simulink model "asbQuadcopters_SiFi"  (Simulink 9.1)
settings: Solver=VariableStepAuto  StartTime=0.0  StopTime=TFinal  RelTol=1e-3
values from neighbouring files (symbols this model uses):
  Controller =     [data_set.mat]
  Estimator =     [data_set.mat]
  g = 9.81    [data_set.mat]
  init =     [data_set.mat]
  rho = 1.184    [data_set.mat]
  sensorCalibrationData = [0.09 -0.06 -9.473 -0.0095 -0.0075 0.0015 101270.95 0.2]    [data_set.mat]
  Sensors =     [data_set.mat]
  States =     [data_set.mat]
  takeOffDuration = 1    [data_set.mat]
  Ts = 0.005    [data_set.mat]
  Vehicle =     [data_set.mat]
undefined symbols (not defined in the file or in its folder): DiscIntNeverNeededParam, Discrete, Earth, ft, m, s, sigbuilder_block, Time, WGS84
libraries: simulink x39, aerolibconvert2 x4, sharedutil x3, ctrlSharedLib x3, sharedtransform x3, shared6dof x1, aerolibasang x1, aerolibtransform2 x1, aerolibnav x1, aerolibanimutils x1
(part 2 of 3)

== system asbQuadcopters_SiFi/FCS/State Estimator/EstimatorXYPosition ==
  opticalFlow_datin : Inport
  controlModePosVSOrient_flagin : Inport  Port=2
  usePosVIS_flagin : Inport  Port=3
  posVIS_datin : Inport  Port=4
  sensorIMU_datin : Inport  Port=5
  Z_estimin : Inport  Port=6
  dz_estimin : Inport  Port=7
  orient_estimin : Inport  Port=8
  EstimatorVelocity : Subsystem
  EstimatorXYPosition : Subsystem
  XY_estimout : Outport
  dxy_estimout : Outport  Port=2
  wires:
  EstimatorXYPosition/1(XY_estimout) -> XY_estimout/1
  usePosVIS_flagin/1 -> EstimatorXYPosition/6(usePosVIS_flagin)
  posVIS_datin/1 -> EstimatorXYPosition/5(posVIS_datin)
  dz_estimin/1 -> EstimatorXYPosition/4(dz_estimin)
  controlModePosVSOrient_flagin/1 -> EstimatorXYPosition/3(controlModePosVSOrient_flagin)
  Z_estimin/1 -> EstimatorVelocity/2(Z_estimin)
  sensorIMU_datin/1 -> EstimatorVelocity/3(sensorIMU_datin)
  opticalFlow_datin/1 -> EstimatorVelocity/1(opticalFlow_datin)
  EstimatorVelocity/1(dxy_estimout) -> dxy_estimout/1, EstimatorXYPosition/1(dxy_estimin)
  orient_estimin/1 -> EstimatorXYPosition/2(orient_estimin), EstimatorVelocity/4(orient_estimin)

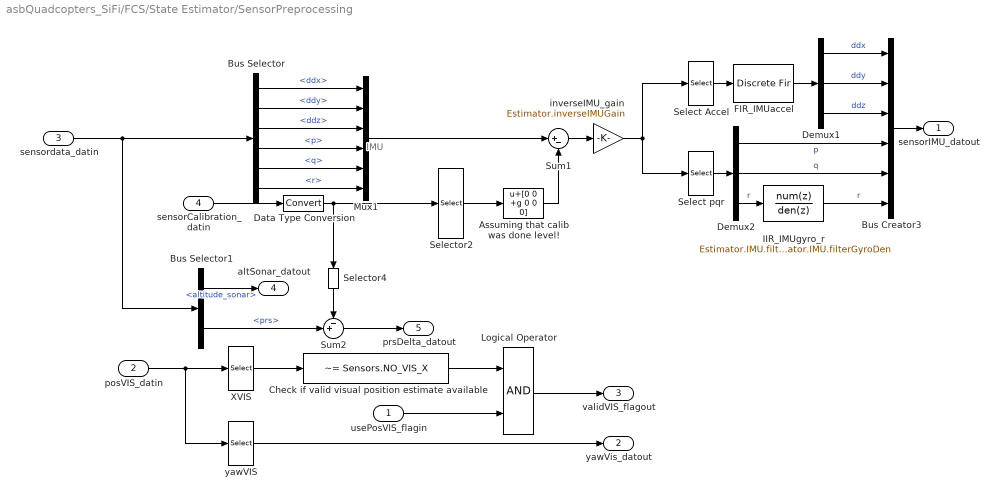
== system asbQuadcopters_SiFi/FCS/State Estimator/SensorPreprocessing ==
  note: IMU
  usePosVIS_flagin : Inport
  posVIS_datin : Inport  Port=2
  sensordata_datin : Inport  Port=3
  sensorCalibration_datin : Inport  Port=4
  Assuming that calib was done level! : Bias  Bias=[0 0 +g 0 0 0]
  Bus Creator3 : BusCreator  Inputs=6
  Bus Selector : BusSelector  OutputSignals=ddx,ddy,ddz,p,q,r
  Bus Selector1 : BusSelector  OutputSignals=altitude_sonar,prs
  Check if valid visual position estimate available : simulink/Logic and Bit Operations/Compare To Constant  relop=~=  const=Sensors.NO_VIS_X  OutDataTypeStr=boolean
  Data Type Conversion : DataTypeConversion
  Demux1 : Demux  Outputs=3
  Demux2 : Demux  Outputs=3
  FIR_IMUaccel : DiscreteFir  Coefficients=Estimator.IMU.filterAccel.Coefficients
  IIR_IMUgyro_r : DiscreteFilter  Numerator=Estimator.IMU.filterGyroNum  Denominator=Estimator.IMU.filterGyroDen
  Logical Operator : Logic  AllPortsSameDT=off  OutDataTypeStr=boolean
  Mux1 : Mux  Inputs=6
  Select Accel : Selector  InputPortWidth=6  IndexOptions=Index vector (dialog)  Indices=[1 2 3]  OutputSizes=1
  Select pqr : Selector  InputPortWidth=6  IndexOptions=Index vector (dialog)  Indices=[4 5 6]  OutputSizes=1
  Selector2 : Selector  InputPortWidth=8  IndexOptions=Index vector (dialog)  Indices=[1:6]  OutputSizes=1
  Selector4 : Selector  InputPortWidth=8  IndexOptions=Index vector (dialog)  Indices=[7]  OutputSizes=1
  Sum1 : Sum  Inputs=|+-
  Sum2 : Sum  Inputs=-+|
  XVIS : Selector  InputPortWidth=4  IndexOptions=Index vector (dialog)  Indices=1  OutputSizes=1
  inverseIMU_gain : Gain  Gain=Estimator.inverseIMUGain  ParamDataTypeStr=single  OutDataTypeStr=single
  yawVIS : Selector  InputPortWidth=4  IndexOptions=Index vector (dialog)  Indices=4  OutputSizes=1
  sensorIMU_datout : Outport
  yawVis_datout : Outport  Port=2
  validVIS_flagout : Outport  Port=3
  altSonar_datout : Outport  Port=4
  prsDelta_datout : Outport  Port=5
  wires:
  Select pqr/1 -> Demux2/1
  Assuming that calib was done level!/1 -> Sum1/2
  usePosVIS_flagin/1 -> Logical Operator/2
  Check if valid visual position estimate available/1 -> Logical Operator/1
  Logical Operator/1 -> validVIS_flagout/1
  yawVIS/1 -> yawVis_datout/1
  XVIS/1 -> Check if valid visual position estimate available/1
  Mux1/1 -> Sum1/1
  Sum2/1 -> prsDelta_datout/1
  Bus Selector1/2 -> Sum2/2  "<prs>"
  Selector4/1 -> Sum2/1
  Bus Selector1/1 -> altSonar_datout/1  "<altitude_sonar>"
  sensordata_datin/1 -> Bus Selector1/1, Bus Selector/1
  Bus Selector/6 -> Mux1/6  "<r>"
  Bus Selector/5 -> Mux1/5  "<q>"
  Bus Selector/4 -> Mux1/4  "<p>"
  Bus Selector/3 -> Mux1/3  "<ddz>"
  Bus Selector/2 -> Mux1/2  "<ddy>"
  Bus Selector/1 -> Mux1/1  "<ddx>"
  sensorCalibration_datin/1 -> Data Type Conversion/1
  IIR_IMUgyro_r/1 -> Bus Creator3/6  "r"
  Demux2/3 -> IIR_IMUgyro_r/1  "r"
  FIR_IMUaccel/1 -> Demux1/1
  Select Accel/1 -> FIR_IMUaccel/1
  inverseIMU_gain/1 -> Select Accel/1, Select pqr/1
  Demux2/2 -> Bus Creator3/5  "q"
  Demux2/1 -> Bus Creator3/4  "p"
  Selector2/1 -> Assuming that calib was done level!/1
  Sum1/1 -> inverseIMU_gain/1
  Demux1/3 -> Bus Creator3/3  "ddz"
  Demux1/2 -> Bus Creator3/2  "ddy"
  Demux1/1 -> Bus Creator3/1  "ddx"
  Bus Creator3/1 -> sensorIMU_datout/1
  posVIS_datin/1 -> XVIS/1, yawVIS/1
  Data Type Conversion/1 -> Selector2/1, Selector4/1

== system asbQuadcopters_SiFi/FCS/controller/Attitude ==
  note: ATTITUDE
  refAttitude : Inport
  states_estim : Inport  Port=2
  Add : Sum  Inputs=+-
  Bus Selector3 : BusSelector  OutputSignals=pitch,roll
  Bus Selector4 : BusSelector  OutputSignals=q,p
  D_pr : Gain  Gain=[0.002;0.003]
  Delay : Delay  DelayLength=1  InitialCondition=0
  Demux : Demux  Outputs=2
  Discrete-Time Integrator : DiscreteIntegrator  SampleTime=Ts  LimitOutput=on  UpperSaturationLimit=2  LowerSaturationLimit=-2  ICPrevOutput=DiscIntNeverNeededParam  ICPrevScaledInput=DiscIntNeverNeededParam
  I_pr : Gain  Gain=0.01
  Mux : Mux  Inputs=2
  Mux1 : Mux  Inputs=2
  P_pr : Gain  Gain=[0.013;0.02]
  Sum16 : Sum  Inputs=++-  AccumDataTypeStr=single  OutDataTypeStr=single  SaturateOnIntegerOverflow=on
  Sum19 : Sum  Inputs=+-|
  antiWU_Gain : Gain  Gain=0.001
  tau_pitch : Outport
  tau_roll : Outport  Port=2
  wires:
  Sum16/1 -> Demux/1  "P_pr"
  antiWU_Gain/1 -> Add/2
  Add/1 -> Discrete-Time Integrator/1
  Bus Selector3/1 -> Mux/1  "<pitch>"
  Bus Selector4/1 -> Mux1/1  "<q>"
  P_pr/1 -> Sum16/1
  I_pr/1 -> Sum16/2
  Sum19/1 -> Add/1, P_pr/1  "pitch/roll error"
  Discrete-Time Integrator/1 -> Delay/1, I_pr/1
  Delay/1 -> antiWU_Gain/1
  Demux/1 -> tau_pitch/1  "tau_pitch"
  Demux/2 -> tau_roll/1
  D_pr/1 -> Sum16/3
  states_estim/1 -> Bus Selector3/1, Bus Selector4/1
  refAttitude/1 -> Sum19/1
  Mux/1 -> Sum19/2
  Bus Selector3/2 -> Mux/2  "<roll>"
  Mux1/1 -> D_pr/1
  Bus Selector4/2 -> Mux1/2  "<p>"

== system asbQuadcopters_SiFi/FCS/controller/ControlMixer ==
  tau_pitch : Inport
  tau_roll : Inport  Port=2
  tau_yaw : Inport  Port=3
  totalThrust : Inport  Port=4
  Mux2 : Mux
  Product : Product  Multiplication=Matrix(*)  RndMeth=Zero
  TorqueTotalThrustToThrustPerMotor : Constant  Value=Controller.Q2Ts  OutDataTypeStr=single
  thrusts_refout : Outport
  wires:
  Product/1 -> thrusts_refout/1
  tau_roll/1 -> Mux2/4
  tau_pitch/1 -> Mux2/3
  tau_yaw/1 -> Mux2/2
  totalThrust/1 -> Mux2/1
  TorqueTotalThrustToThrustPerMotor/1 -> Product/1
  Mux2/1 -> Product/2

== system asbQuadcopters_SiFi/FCS/controller/XY-to-reference-orientation ==
  posXY : Inport
  states_estim : Inport  Port=2
  yaw : Inport  Port=3
  Bus Selector1 : BusSelector  OutputSignals=X,Y
  Bus Selector2 : BusSelector  OutputSignals=dx,dy
  D_xy : Gain  Gain=[0.1, -0.1]  ParamDataTypeStr=single  OutDataTypeStr=single  SaturateOnIntegerOverflow=on
  Gain : Gain  Gain=-1
  Matrix Concatenate : Concatenate  Mode=Multidimensional array  ConcatenateDimension=2
  Mux : Mux  Inputs=2
  Mux1 : Mux  Inputs=2
  P_xy : Gain  Gain=[-0.24,0.24]  ParamDataTypeStr=single  OutDataTypeStr=single  SaturateOnIntegerOverflow=on
  Product : Product  Multiplication=Matrix(*)  OutDataTypeStr=single  RndMeth=Zero
  Saturation : Saturate  UpperLimit=3  LowerLimit=-3  OutDataTypeStr=single
  Sum17 : Sum  Inputs=+-|  AccumDataTypeStr=single
  Sum18 : Sum  Inputs=|++  AccumDataTypeStr=single  OutDataTypeStr=single  SaturateOnIntegerOverflow=on
  Trigonometric Function : Trigonometry  Operator=sincos
  Vector Concatenate : Concatenate
  Vector Concatenate1 : Concatenate
  pitch_roll_cmd : Outport
  wires:
  yaw/1 -> Trigonometric Function/1
  Saturation/1 -> P_xy/1
  P_xy/1 -> Sum18/1
  Sum17/1 -> Product/2  "XY error"
  posXY/1 -> Sum17/1
  Bus Selector2/1 -> Mux1/1  "<dx>"
  states_estim/1 -> Bus Selector1/1, Bus Selector2/1
  Sum18/1 -> pitch_roll_cmd/1  "pitch/roll cmd"
  D_xy/1 -> Sum18/2
  Bus Selector1/1 -> Mux/1  "<X>"
  Product/1 -> Saturation/1
  Trigonometric Function/1 -> Gain/1, Vector Concatenate1/1
  Trigonometric Function/2 -> Vector Concatenate1/2, Vector Concatenate/1
  Gain/1 -> Vector Concatenate/2
  Vector Concatenate/1 -> Matrix Concatenate/1
  Vector Concatenate1/1 -> Matrix Concatenate/2
  Matrix Concatenate/1 -> Product/1
  Bus Selector1/2 -> Mux/2  "<Y>"
  Mux/1 -> Sum17/2
  Mux1/1 -> D_xy/1
  Bus Selector2/2 -> Mux1/2  "<dy>"

== system asbQuadcopters_SiFi/FCS/controller/Yaw ==
  yaw_ref : Inport
  states_estim : Inport  Port=2
  Bus Selector5 : BusSelector  OutputSignals=yaw,r
  D_yaw : Gain  Gain=0.3*0.004
  P_yaw : Gain  Gain=0.004  ParamDataTypeStr=single  OutDataTypeStr=single
  Sum1 : Sum  Inputs=+-|  AccumDataTypeStr=single  OutDataTypeStr=single  SaturateOnIntegerOverflow=on
  Sum2 : Sum  Inputs=|+-
  yaw : Outport
  tau_yaw : Outport  Port=2
  wires:
  D_yaw/1 -> Sum2/2
  P_yaw/1 -> Sum2/1
  Bus Selector5/2 -> D_yaw/1  "<r>"
  Sum1/1 -> P_yaw/1
  states_estim/1 -> Bus Selector5/1
  Sum2/1 -> tau_yaw/1
  Bus Selector5/1 -> yaw/1, Sum1/2  "<yaw>"
  yaw_ref/1 -> Sum1/1

== system asbQuadcopters_SiFi/FCS/controller/gravity feedforward/equilibrium thrust ==
  note: ALTITUDE
  states_estim : Inport
  PosZ : Inport  Port=2
  takeoff_flag : Inport  Port=3
  Bus Selector6 : BusSelector  OutputSignals=Z,dz
  D_z : Gain  Gain=0.3  ParamDataTypeStr=single  OutDataTypeStr=single  SaturateOnIntegerOverflow=on
  P_z : Gain  Gain=0.8  ParamDataTypeStr=single  OutDataTypeStr=single  SaturateOnIntegerOverflow=on
  SaturationThrust : Saturate  UpperLimit=4*Controller.totalThrustMaxRelative*Controller.motorsThrustPerMotorMax  LowerLimit=-4*Controller.totalThrustMaxRelative*Controller.motorsThrustPerMotorMax  OutDataTypeStr=single
  Sum15 : Sum  Inputs=|+-  AccumDataTypeStr=single  OutDataTypeStr=single  SaturateOnIntegerOverflow=on
  Sum3 : Sum  Inputs=+-|  AccumDataTypeStr=single  OutDataTypeStr=single  SaturateOnIntegerOverflow=on
  Sum4 : Sum  Inputs=++|  AccumDataTypeStr=single  OutDataTypeStr=single  SaturateOnIntegerOverflow=on
  TakeoffOrControl_Switch : Switch  Criteria=u2 > Threshold
  takeoff_gain : Gain  Gain=Controller.takeoffGain  ParamDataTypeStr=single  OutDataTypeStr=single  SaturateOnIntegerOverflow=on
  w0 : Constant  Value=-g*Vehicle.Airframe.mass  OutDataTypeStr=single  SampleTime=Ts
  altitude_cmd : Outport
  wires:
  Sum3/1 -> P_z/1  "errZ"
  TakeoffOrControl_Switch/1 -> Sum4/2
  Bus Selector6/1 -> Sum3/2  "<Z>"
  Bus Selector6/2 -> D_z/1  "<dz>"
  w0/1 -> Sum4/1, takeoff_gain/1
  D_z/1 -> Sum15/2  "dz"
  takeoff_gain/1 -> TakeoffOrControl_Switch/1
  takeoff_flag/1 -> TakeoffOrControl_Switch/2
  PosZ/1 -> Sum3/1
  P_z/1 -> Sum15/1
  Sum15/1 -> TakeoffOrControl_Switch/3
  Sum4/1 -> SaturationThrust/1
  SaturationThrust/1 -> altitude_cmd/1
  states_estim/1 -> Bus Selector6/1

== system asbQuadcopters_SiFi/FCS/controller/thrustsToMotorCommands ==
  thrusts_refin : Inport
  MotorDirections : Gain  Gain=[1 -1 1 -1]
  Saturation5 : Saturate  UpperLimit=Vehicle.Motor.maxLimit  LowerLimit=Vehicle.Motor.minLimit
  ThrustToMotorCommand : Gain  Gain=-Vehicle.Motor.thrustToMotorCommand
  motors_cmdout : Outport
  wires:
  Saturation5/1 -> MotorDirections/1
  MotorDirections/1 -> motors_cmdout/1
  ThrustToMotorCommand/1 -> Saturation5/1
  thrusts_refin/1 -> ThrustToMotorCommand/1

== system asbQuadcopters_SiFi/Sensor/Sensor System/Camera ==
  states : Inport
  Add1 : Sum
  Bus Selector1 : BusSelector  OutputSignals=V_ned
  Bus Selector3 : BusSelector  OutputSignals=X_ned
  Bus Selector4 : BusSelector  OutputSignals=Omega_body
  Data Type Conversion : DataTypeConversion  OutDataTypeStr=single
  Demux4 : Demux  Outputs=2
  Gain1 : Gain  Gain=0.8*[-1,1]
  Gain2 : Gain  Gain=-1
  Mux7 : Mux  Inputs=2
  Mux8 : Mux  Inputs=2
  Product : Product
  Product1 : Product
  Reshape : Reshape
  Select dx,dy : Selector  InputPortWidth=3  IndexOptions=Index vector (dialog)  Indices=[1 2]  OutputSizes=1
  Select dx,dy1 : Selector  InputPortWidth=3  IndexOptions=Index vector (dialog)  Indices=[1 2]  OutputSizes=1
  Select dz : Selector  InputPortWidth=3  IndexOptions=Index vector (dialog)  Indices=3  OutputSizes=1
  Select dz1 : Selector  InputPortWidth=3  IndexOptions=Index vector (dialog)  Indices=3  OutputSizes=1
  SwitchPlanarOpticalFlow : Selector  InputPortWidth=2  IndexOptions=Index vector (dialog)  Indices=[2 1]  OutputSizes=1
  VelocityToOpticalFlow_Gain : Gain  Gain=Sensors.velocityToOpticalFlowGain
  opticalFlow_datout : Outport
  wires:
  Gain1/1 -> Demux4/1
  Data Type Conversion/1 -> opticalFlow_datout/1
  Bus Selector4/1 -> Reshape/1  "<Omega_body>"
  Select dz1/1 -> Gain2/1
  Bus Selector3/1 -> Select dz1/1  "<X_ned>"
  Select dz/1 -> Mux8/2
  Gain2/1 -> Product1/2, Product/2
  Mux8/1 -> VelocityToOpticalFlow_Gain/1
  Demux4/1 -> Product/1
  states/1 -> Bus Selector1/1, Bus Selector4/1, Bus Selector3/1
  Add1/1 -> Mux8/1
  Product/1 -> Mux7/1
  Product1/1 -> Mux7/2
  Demux4/2 -> Product1/1
  Bus Selector1/1 -> Select dz/1, Select dx,dy/1  "<V_ned>"
  Reshape/1 -> Select dx,dy1/1
  Select dx,dy1/1 -> Gain1/1
  Select dx,dy/1 -> Add1/1
  Mux7/1 -> SwitchPlanarOpticalFlow/1
  VelocityToOpticalFlow_Gain/1 -> Data Type Conversion/1
  SwitchPlanarOpticalFlow/1 -> Add1/2

== system asbQuadcopters_SiFi/Sensor/Sensor System/IMU_Pressure ==
  States : Inport
  Environment : Inport  Port=2
  Assumes takeoff was level1 : Bias  Bias=Sensors.altToPrsBias
  Bus Selector : BusSelector  OutputSignals=Accel_body,Omega_body,dOmega_body,DCM_be,X_ned
  Bus Selector1 : BusSelector  OutputSignals=Gravity_ned
  CG location : Constant  Value=Sensors.IMU.cg
  Data Type Conversion{,1..4} (5 alike) : DataTypeConversion  OutDataTypeStr=single
  Demux : Demux  Outputs=3
  Demux2 : Demux  Outputs=3
  HAL_acquisition_creator : Subsystem
  Mux : Mux  Inputs=8
  Product : Product  Multiplication=Matrix(*)
  Saturation : Saturate  UpperLimit=inf  LowerLimit=Sensors.altSensorMin  OutDataTypeStr=single
  Selector2 : Selector  InputPortWidth=3  IndexOptions=Index vector (dialog)  Indices=[3]  OutputSizes=1
  Three-axis Inertial Measurement Unit : aerolibnav/Three-axis Inertial Measurement Unit  units=Metric (MKS)  imu=Sensors.IMU.location  i_Ts=Ts  dtype_a=off  w_a=.7  z_a=.2  a_sf_cc=Sensors.IMU.accScaleCross  a_bias=Sensors.IMU.accBias  a_sat=Sensors.IMU.accLimits  dtype_g=off  w_g=.7  z_g=.2  g_sf_cc=Sensors.IMU.gyroScaleCross  g_bias=Sensors.IMU.gyroBias  g_sens=Sensors.IMU.gyroGBias  g_sat=Sensors.IMU.gyroLimits  i_rand=on  i_seeds=Sensors.IMU.noiseSeeds  i_pow=Sensors.IMU.noisePower
  altToprs_gain : Gain  Gain=Sensors.altToPrsGain  ParamDataTypeStr=single  OutDataTypeStr=single
  altToprs_gain1 : Gain  Gain=-1  ParamDataTypeStr=single  OutDataTypeStr=single
  sensordata_datout : Outport  OutDataTypeStr=Bus: HAL_acquisition_t
  wires:
  altToprs_gain/1 -> Assumes takeoff was level1/1  "prs"
  Demux/3 -> Mux/3  "ddz"
  Demux2/3 -> Mux/6  "r"
  Demux2/1 -> Mux/4  "p"
  Data Type Conversion1/1 -> HAL_acquisition_creator/1(sensors)
  Demux/1 -> Mux/1  "ddx"
  Data Type Conversion2/1 -> Demux2/1
  Three-axis Inertial Measurement Unit/2 -> Data Type Conversion2/1
  Demux/2 -> Mux/2  "ddy"
  Saturation/1 -> Data Type Conversion3/1  "altitude_sonar"
  Environment/1 -> Bus Selector1/1
  CG location/1 -> Three-axis Inertial Measurement Unit/4
  HAL_acquisition_creator/1(HAL_acquisition_t) -> sensordata_datout/1
  Bus Selector/1 -> Three-axis Inertial Measurement Unit/1  "<Accel_body>"
  altToprs_gain1/1 -> Saturation/1
  Bus Selector/3 -> Three-axis Inertial Measurement Unit/3  "<dOmega_body>"
  Bus Selector1/1 -> Product/2  "<Gravity_ned>"
  Bus Selector/4 -> Product/1  "<DCM_be>"
  Data Type Conversion3/1 -> Mux/7
  Bus Selector/2 -> Three-axis Inertial Measurement Unit/2  "<Omega_body>"
  Assumes takeoff was level1/1 -> Data Type Conversion4/1
  Product/1 -> Three-axis Inertial Measurement Unit/5
  Mux/1 -> Data Type Conversion1/1
  Data Type Conversion/1 -> Demux/1
  Data Type Conversion4/1 -> Mux/8
  States/1 -> Bus Selector/1
  Selector2/1 -> altToprs_gain/1, altToprs_gain1/1
  Bus Selector/5 -> Selector2/1  "<X_ned>"
  Demux2/2 -> Mux/5  "q"
  Three-axis Inertial Measurement Unit/1 -> Data Type Conversion/1

== system asbQuadcopters_SiFi/Airframe/AC model/Drag Calculation/Drag Calc ==
  Density : Inport  Unit=kg/m^3
  vel : Inport  Port=2  Unit=m/s
  Dynamic Pressure : aerolibasang/Dynamic Pressure
  Gain : Gain  Gain=[.25 .25]
  Mux1 : Mux  Inputs=2
  Product : Product  Inputs=3  RndMeth=Zero
  diameter : Constant  Value=Vehicle.Airframe.diameter  SampleTime=0
  dragCoeff : Constant  Value=Vehicle.Airframe.Cdx  SampleTime=0
  drag : Outport  Unit=N
  wires:
  Product/1 -> drag/1
  dragCoeff/1 -> Product/3  "Cd"
  Dynamic Pressure/1 -> Product/1  "q"
  diameter/1 -> Gain/1, Mux1/2
  Mux1/1 -> Product/2  "S"
  Gain/1 -> Mux1/1
  vel/1 -> Dynamic Pressure/1
  Density/1 -> Dynamic Pressure/2

== system asbQuadcopters_SiFi/Airframe/AC model/Motor Forces and Torques/For Each Subsystem ==
  Vb : Inport  PortDimensions=3
  rho : Inport  Port=2  PortDimensions=1
  Omega : Inport  Port=3
  w : Inport  Port=4  Partition=on  PartitionDimension=2  PartitionWidth=1  PartitionOffset=0
  D : Inport  Port=5  Partition=on  PartitionDimension=2  PartitionWidth=1  PartitionOffset=0
  For Each : ForEach  DisableCoverage=on  IndexMode=One-based
  Subsystem : Subsystem
  Forces : Outport  ConcatenationDimension=2
  Moments : Outport  Port=2  ConcatenationDimension=2
  wires:
  Vb/1 -> Subsystem/1(Vb)
  Omega/1 -> Subsystem/2(pqr)
  rho/1 -> Subsystem/3(rho)
  w/1 -> Subsystem/4(w)
  D/1 -> Subsystem/5(Arm)
  Subsystem/1(Fxyz) -> Forces/1
  Subsystem/2(Mxyz) -> Moments/1

== system asbQuadcopters_SiFi/Airframe/AC model/Motor Forces and Torques/MotorsToW ==
  motors_datin : Inport
  Motordirections : Gain  Gain=[1 -1 1 -1]  ParamDataTypeStr=single  OutDataTypeStr=Inherit: Inherit via back propagation  SaturateOnIntegerOverflow=on
  Motordirections1 : Gain  Gain=[1 -1 1 -1]  ParamDataTypeStr=single  OutDataTypeStr=Inherit: Inherit via back propagation  SaturateOnIntegerOverflow=on
  Saturation5 : Saturate  UpperLimit=Vehicle.Motor.maxLimit  LowerLimit=Vehicle.Motor.minLimit  OutDataTypeStr=Inherit: Inherit via back propagation
  Signed Sqrt : Sqrt  Operator=signedSqrt  OutDataTypeStr=Inherit: Inherit via back propagation  SaturateOnIntegerOverflow=on
  motorsToW2_Gain : Gain  Gain=Vehicle.Motor.commandToW2Gain  ParamDataTypeStr=single  OutDataTypeStr=Inherit: Inherit via back propagation  SaturateOnIntegerOverflow=on
  omegas_datout : Outport
  wires:
  motorsToW2_Gain/1 -> Signed Sqrt/1
  Motordirections/1 -> Saturation5/1
  Saturation5/1 -> Motordirections1/1
  Motordirections1/1 -> motorsToW2_Gain/1
  Signed Sqrt/1 -> omegas_datout/1
  motors_datin/1 -> Motordirections/1

== system asbQuadcopters_SiFi/FCS/State Estimator/Complementary Filter/If Action Subsystem ==
  rpy : Inport
  accel : Inport  Port=2
  Action Port : ActionPort  ActionType=then
  Demux : Demux  Outputs=3
  Demux1 : Demux  Outputs=3
  Divide : Product  Inputs=*/
  Gain : Gain  Gain=1-Estimator.gyroAngleUpdateAccWeight
  Gain1 : Gain  Gain=Estimator.gyroAngleUpdateAccWeight
  Gain2 : Gain  Gain=1/g
  Gain3 : Gain  Gain=Estimator.gyroAngleUpdateAccWeight
  Gain4 : Gain  Gain=1-Estimator.gyroAngleUpdateAccWeight
  Mux : Mux  Inputs=2
  Sum : Sum  Inputs=|++
  Sum1 : Sum  Inputs=|++
  Terminator1 : Terminator
  Trigonometric Function : Trigonometry  Operator=atan
  Trigonometric Function1 : Trigonometry  Operator=asin
  pitch,roll : Outport
  wires:
  accel/1 -> Demux/1
  Demux/2 -> Divide/1
  Demux/3 -> Divide/2
  Divide/1 -> Trigonometric Function/1
  Gain/1 -> Sum/1
  Trigonometric Function/1 -> Gain1/1
  Mux/1 -> pitch,roll/1
  Gain2/1 -> Trigonometric Function1/1
  Trigonometric Function1/1 -> Gain3/1
  Gain4/1 -> Sum1/1
  Gain3/1 -> Sum1/2
  Sum1/1 -> Mux/1
  Sum/1 -> Mux/2
  rpy/1 -> Demux1/1
  Demux1/1 -> Gain/1
  Demux1/2 -> Gain4/1
  Demux/1 -> Gain2/1
  Demux1/3 -> Terminator1/1
  Gain1/1 -> Sum/2

== system asbQuadcopters_SiFi/FCS/State Estimator/Complementary Filter/If Action Subsystem1 ==
  rpy : Inport
  yawVis : Inport  Port=2
  Action Port : ActionPort  ActionType=then
  Gain : Gain  Gain=1-Estimator.gyroAngleUpdateVisWeight
  Gain1 : Gain  Gain=Estimator.gyroAngleUpdateVisWeight
  Selector4 : Selector  InputPortWidth=3  IndexOptions=Index vector (dialog)  Indices=[3]  OutputSizes=1
  Sum : Sum  Inputs=|++
  yaw : Outport
  wires:
  rpy/1 -> Selector4/1
  Selector4/1 -> Gain/1
  yawVis/1 -> Gain1/1
  Gain/1 -> Sum/1
  Gain1/1 -> Sum/2
  Sum/1 -> yaw/1

== system asbQuadcopters_SiFi/FCS/State Estimator/Complementary Filter/If Action Subsystem2 ==
  prin : Inport
  Action Port : ActionPort  ActionType=else
  prout : Outport
  wires:
  prin/1 -> prout/1

== system asbQuadcopters_SiFi/FCS/State Estimator/Complementary Filter/If Action Subsystem3 ==
  yawin : Inport
  Action Port : ActionPort  ActionType=else
  yout : Outport
  wires:
  yawin/1 -> yout/1

== system asbQuadcopters_SiFi/FCS/State Estimator/Complementary Filter/Wbe ==
  rpy : Inport  OutDataTypeStr=single
  Constant : Constant  Value=single(0)
  Create 3x3 Matrix : sharedutil/Create 3x3 Matrix  aMode=aMode
  Divide : Product  Inputs=*/
  Gain : Gain  Gain=-1
  Product{1..4} (4 alike) : Product
  Selector : Selector  InputPortWidth=3  IndexOptions=Index vector (dialog)  Indices=[1]  OutputSizes=1
  Selector1 : Selector  InputPortWidth=3  IndexOptions=Index vector (dialog)  Indices=[1]  OutputSizes=1
  Selector2 : Selector  InputPortWidth=3  IndexOptions=Index vector (dialog)  Indices=[2]  OutputSizes=1
  Selector3 : Selector  InputPortWidth=3  IndexOptions=Index vector (dialog)  Indices=[2]  OutputSizes=1
  Trigonometric Function : Trigonometry  Operator=sincos
  Wbe : Outport
  wires:
  Create 3x3 Matrix/1 -> Divide/1
  Product3/1 -> Create 3x3 Matrix/8
  Trigonometric Function/2 -> Selector1/1, Selector2/1
  Selector3/1 -> Product4/2, Product3/2
  Selector1/1 -> Product4/1, Product1/1, Create 3x3 Matrix/3
  Trigonometric Function/1 -> Selector3/1, Selector/1
  Product1/1 -> Create 3x3 Matrix/5
  Product2/1 -> Create 3x3 Matrix/6
  Selector2/1 -> Divide/2, Create 3x3 Matrix/7, Product2/1, Product1/2
  Gain/1 -> Product2/2
  Product4/1 -> Create 3x3 Matrix/9
  Constant/1 -> Create 3x3 Matrix/4, Create 3x3 Matrix/1
  Divide/1 -> Wbe/1
  rpy/1 -> Trigonometric Function/1
  Selector/1 -> Product3/1, Gain/1, Create 3x3 Matrix/2

== system asbQuadcopters_SiFi/FCS/State Estimator/EstimatorAltitude/OutlierHandling ==
  altSonar_datin : Inport
  altPrs_datin : Inport  Port=2
  Z_estimin : Inport  Port=3
  Absestdiff : Abs
  Absestdiff1 : Abs
  Absestdiff2 : Abs
  Add : Sum  Inputs=-+
  Add1 : Sum  Inputs=-+
  Add2 : Sum  Inputs=-+
  SaturationSonar : Saturate  UpperLimit=-Sensors.altSensorMin  LowerLimit=-inf
  check for min altitude : simulink/Logic and Bit Operations/Compare To Constant  relop=<  const=-Sensors.altSensorMin  OutDataTypeStr=boolean
  currentEstimateVeryOffFromPressure : simulink/Logic and Bit Operations/Compare To Constant  relop=>=  const=Estimator.alt.deltaPrsToCurrentThreshold  OutDataTypeStr=boolean
  currentStateVeryOffsonarflt : simulink/Logic and Bit Operations/Compare To Constant  relop=>=  const=Estimator.alt.deltaSonarToFilteredThreshold  OutDataTypeStr=boolean
  findingoutliers : Logic  AllPortsSameDT=off  OutDataTypeStr=boolean
  newupdateneeded : Logic  AllPortsSameDT=off  OutDataTypeStr=boolean
  nicemeasurementor newupdateneeded : Logic  Operator=OR  AllPortsSameDT=off  OutDataTypeStr=boolean
  outlierJump : simulink/Logic and Bit Operations/Compare To Constant  relop=<=  const=Estimator.alt.deltaSonarToCurrentMax  OutDataTypeStr=boolean
  pressureFilter_IIR : DiscreteFilter  Numerator=Estimator.alt.filterPrsNum  Denominator=Estimator.alt.filterPrsDen
  soonarFilter_IIR : DiscreteFilter  Numerator=Estimator.alt.filterSonarNum  Denominator=Estimator.alt.filterSonarDen
  enableKFmeasupdate_flagout : Outport
  wires:
  Add1/1 -> Absestdiff1/1
  nicemeasurementor newupdateneeded/1 -> enableKFmeasupdate_flagout/1
  findingoutliers/1 -> nicemeasurementor newupdateneeded/1
  check for min altitude/1 -> findingoutliers/2
  outlierJump/1 -> findingoutliers/1
  SaturationSonar/1 -> Add/1
  Absestdiff/1 -> outlierJump/1
  Add/1 -> Absestdiff/1
  newupdateneeded/1 -> nicemeasurementor newupdateneeded/2
  Absestdiff2/1 -> currentStateVeryOffsonarflt/1
  altSonar_datin/1 -> SaturationSonar/1, soonarFilter_IIR/1, check for min altitude/1
  currentEstimateVeryOffFromPressure/1 -> newupdateneeded/1
  Z_estimin/1 -> Add1/1, Add2/1, Add/2
  Add2/1 -> Absestdiff2/1
  currentStateVeryOffsonarflt/1 -> newupdateneeded/2
  pressureFilter_IIR/1 -> Add1/2
  altPrs_datin/1 -> pressureFilter_IIR/1
  soonarFilter_IIR/1 -> Add2/2
  Absestdiff1/1 -> currentEstimateVeryOffFromPressure/1

== system asbQuadcopters_SiFi/FCS/State Estimator/EstimatorXYPosition/EstimatorVelocity ==
  opticalFlow_datin : Inport
  Z_estimin : Inport  Port=2  SampleTime=Ts
  sensorIMU_datin : Inport  Port=3
  orient_estimin : Inport  Port=4
  AccelerationHandling : Subsystem
  DataHandling : Subsystem
  Delay : Delay  DelayLength=1  InitialCondition=0
  KalmanFilter_dxdy : ctrlSharedLib/Kalman Filter  TimeDomain=Discrete-Time  UseCurrentEstimator=on  ModelSource=Individual A, B, C, D matrices  ModelSourceVariable=ss(0.95,1,1,0,1)  A=eye(2)  B=Ts*eye(2)  C=eye(2)  D=0  NumberOfStates=1  NumberOfInputs=1  NumberOfOutputs=1  InitialEstimateSource=Dialog  X0=0  P0=10  UseK=off  UseGH=on  NumberOfProcessNoiseInputs=1  G=Estimator.pos.kfVelo.G  TimeInvariantG=on  H=Estimator.pos.kfVelo.H  TimeInvariantH=on  Q=Estimator.pos.kfVelo.Q  TimeInvariantQ=on  R=Estimator.pos.kfVelo.R  TimeInvariantR=on  N=Estimator.pos.kfVelo.N  TimeInvariantN=on  AddInputPort=on  AddEnablePort=on  OutputEstimatedY=off  OutputP=off  Ts=-1
      settings: SourceProductBaseCode=CT
  Select dxy : Selector  InputPortWidth=3  IndexOptions=Index vector (dialog)  Indices=[1 2]  OutputSizes=1
  opticalFlowToVelocity_gain : Gain  Gain=Estimator.pos.opticalFlowToVelocityGain
  dxy_estimout : Outport
  wires:
  Delay/1 -> DataHandling/5(dxyOF_datin)
  Z_estimin/1 -> DataHandling/1(Z_estimin), AccelerationHandling/4(Z_estimin)
  KalmanFilter_dxdy/1 -> dxy_estimout/1, Delay/1
  opticalFlowToVelocity_gain/1 -> Select dxy/1
  opticalFlow_datin/1 -> opticalFlowToVelocity_gain/1
  sensorIMU_datin/1 -> AccelerationHandling/2(sensorIMU_datin), DataHandling/3(sensorIMU_datin)
  orient_estimin/1 -> AccelerationHandling/3(orient_estimin), DataHandling/2(orient_estimin)
  Select dxy/1 -> KalmanFilter_dxdy/2, AccelerationHandling/1(dxy_estimin), DataHandling/4(dxy_estimin)
  AccelerationHandling/1(acceleration_world) -> KalmanFilter_dxdy/1
  DataHandling/1(enable_flag) -> KalmanFilter_dxdy/3

== system asbQuadcopters_SiFi/FCS/State Estimator/EstimatorXYPosition/EstimatorXYPosition ==
  note: Switching from orientationControl to Position
      | control reset the current world position estimate
      | (happens when using no markers)
  dxy_estimin : Inport
  orient_estimin : Inport  Port=2  SampleTime=Ts
  controlModePosVSOrient_flagin : Inport  Port=3
  dz_estimin : Inport  Port=4
  posVIS_datin : Inport  Port=5
  usePosVIS_flagin : Inport  Port=6
  Delay : Delay  DelayLength=1  InitialCondition=0
  KalmanFilter_posxy : ctrlSharedLib/Kalman Filter  TimeDomain=Discrete-Time  UseCurrentEstimator=on  ModelSource=Individual A, B, C, D matrices  ModelSourceVariable=ss(0.95,1,1,0,1)  A=eye(2)  B=Ts*eye(2)  C=eye(2)  D=0  NumberOfStates=1  NumberOfInputs=1  NumberOfOutputs=1  InitialEstimateSource=Dialog  X0=[.1 0]  P0=10  UseK=off  UseGH=on  NumberOfProcessNoiseInputs=1  G=Estimator.pos.kfPos.G  TimeInvariantG=on  H=Estimator.pos.kfPos.H  TimeInvariantH=on  Q=Estimator.pos.kfPos.Q  TimeInvariantQ=on  R=Estimator.pos.kfPos.R  TimeInvariantR=on  N=Estimator.pos.kfPos.N  TimeInvariantN=on  AddInputPort=on  AddEnablePort=on  OutputEstimatedY=off  OutputP=off  Ts=-1
      settings: SourceProductBaseCode=CT
  Math Function : Math  Operator=transpose  SaturateOnIntegerOverflow=on
  Mux2 : Mux  Inputs=2
  OutlierHandling : Subsystem
  Product : Product  Multiplication=Matrix(*)
  Rotation Angles to Direction Cosine Matrix : sharedtransform/Rotation Angles to Direction Cosine Matrix  rotationOrder=ZYX  aMode=aMode
      settings: SourceProductBaseCode=AE
  SelectXY : Selector  InputPortWidth=4  IndexOptions=Index vector (dialog)  Indices=[1 2]  OutputSizes=1
  SelectdXY : Selector  InputPortWidth=3  IndexOptions=Index vector (dialog)  Indices=[1 2]  OutputSizes=1
  SimplyIntegrateVelocity : DiscreteIntegrator  ExternalReset=rising  SampleTime=Ts  ICPrevOutput=DiscIntNeverNeededParam  ICPrevScaledInput=DiscIntNeverNeededParam
  UseIPPosSwitch : Switch  Criteria=u2 > Threshold
  XY_estimout : Outport
  wires:
  Delay/1 -> OutlierHandling/3(pos_estim)
  usePosVIS_flagin/1 -> UseIPPosSwitch/2
  UseIPPosSwitch/1 -> XY_estimout/1
  controlModePosVSOrient_flagin/1 -> SimplyIntegrateVelocity/2
  KalmanFilter_posxy/1 -> Delay/1, UseIPPosSwitch/1
  posVIS_datin/1 -> OutlierHandling/2(posVIS_datin), SelectXY/1
  Product/1 -> SelectdXY/1
  Mux2/1 -> Product/2
  dz_estimin/1 -> Mux2/2
  SimplyIntegrateVelocity/1 -> UseIPPosSwitch/3
  dxy_estimin/1 -> Mux2/1
  orient_estimin/1 -> Rotation Angles to Direction Cosine Matrix/1, OutlierHandling/1(orient_estimin)
  Rotation Angles to Direction Cosine Matrix/1 -> Math Function/1
  SelectXY/1 -> KalmanFilter_posxy/2
  OutlierHandling/1(enable_flag) -> KalmanFilter_posxy/3
  SelectdXY/1 -> SimplyIntegrateVelocity/1, KalmanFilter_posxy/1
  Math Function/1 -> Product/1

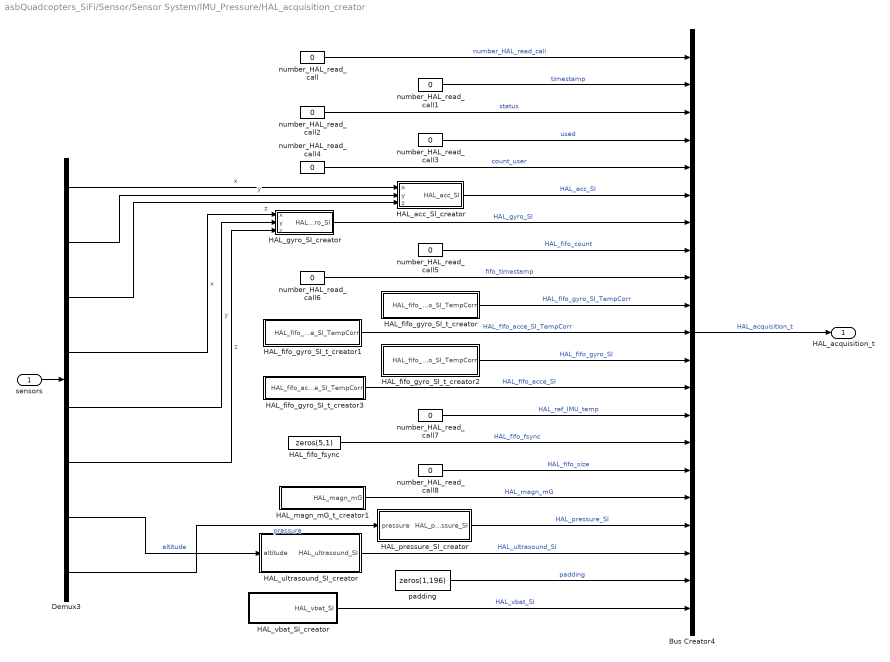
== system asbQuadcopters_SiFi/Sensor/Sensor System/IMU_Pressure/HAL_acquisition_creator ==
  sensors : Inport
  Bus Creator4 : BusCreator  Inputs=21  OutDataTypeStr=Bus: HAL_acquisition_t  NonVirtualBus=on
      settings: InheritFromInputs=off
  Demux3 : Demux  Outputs=8
  HAL_acc_SI_creator : Subsystem
  HAL_fifo_fsync : Constant  Value=zeros(5,1)  OutDataTypeStr=uint8
  HAL_fifo_gyro_SI_t_creator : Subsystem
  HAL_fifo_gyro_SI_t_creator1 : Subsystem
  HAL_fifo_gyro_SI_t_creator2 : Subsystem
  HAL_fifo_gyro_SI_t_creator3 : Subsystem
  HAL_gyro_SI_creator : Subsystem
  HAL_magn_mG_t_creator1 : Subsystem
  HAL_pressure_SI_creator : Subsystem
  HAL_ultrasound_SI_creator : Subsystem
  HAL_vbat_SI_creator : Subsystem
  number_HAL_read_call : Constant  Value=0  OutDataTypeStr=int32
  number_HAL_read_call1 : Constant  Value=0  OutDataTypeStr=uint32
  number_HAL_read_call2 : Constant  Value=0  OutDataTypeStr=uint16
  number_HAL_read_call3 : Constant  Value=0  OutDataTypeStr=uint8
  number_HAL_read_call4 : Constant  Value=0  OutDataTypeStr=uint8
  number_HAL_read_call5 : Constant  Value=0  OutDataTypeStr=uint16
  number_HAL_read_call6 : Constant  Value=0  OutDataTypeStr=uint32
  number_HAL_read_call7 : Constant  Value=0  OutDataTypeStr=single
  number_HAL_read_call8 : Constant  Value=0  OutDataTypeStr=int32
  padding : Constant  Value=zeros(1,196)  OutDataTypeStr=uint8
  HAL_acquisition_t : Outport  OutDataTypeStr=Bus: HAL_acquisition_t
  wires:
  Demux3/4 -> HAL_gyro_SI_creator/1(x)  "x"
  HAL_gyro_SI_creator/1(HAL_gyro_SI) -> Bus Creator4/7  "HAL_gyro_SI"
  Demux3/7 -> HAL_ultrasound_SI_creator/1(altitude)  "altitude"
  HAL_fifo_gyro_SI_t_creator2/1(HAL_fifo_gyro_SI_TempCorr) -> Bus Creator4/12  "HAL_fifo_gyro_SI"
  HAL_magn_mG_t_creator1/1(HAL_magn_mG) -> Bus Creator4/17  "HAL_magn_mG"
  HAL_vbat_SI_creator/1(HAL_vbat_SI) -> Bus Creator4/21  "HAL_vbat_SI"
  sensors/1 -> Demux3/1
  number_HAL_read_call4/1 -> Bus Creator4/5  "count_user"
  Demux3/5 -> HAL_gyro_SI_creator/2(y)  "y"
  number_HAL_read_call8/1 -> Bus Creator4/16  "HAL_fifo_size"
  HAL_fifo_gyro_SI_t_creator1/1(HAL_fifo_acce_SI_TempCorr) -> Bus Creator4/11  "HAL_fifo_acce_SI_TempCorr"
  Demux3/6 -> HAL_gyro_SI_creator/3(z)  "z"
  Demux3/8 -> HAL_pressure_SI_creator/1(pressure)  "pressure"
  number_HAL_read_call/1 -> Bus Creator4/1  "number_HAL_read_call"
  number_HAL_read_call6/1 -> Bus Creator4/9  "fifo_timestamp"
  number_HAL_read_call3/1 -> Bus Creator4/4  "used"
  number_HAL_read_call5/1 -> Bus Creator4/8  "HAL_fifo_count"
  Demux3/2 -> HAL_acc_SI_creator/2(y)  "y"
  number_HAL_read_call2/1 -> Bus Creator4/3  "status"
  Demux3/1 -> HAL_acc_SI_creator/1(x)  "x"
  padding/1 -> Bus Creator4/20  "padding"
  HAL_fifo_fsync/1 -> Bus Creator4/15  "HAL_fifo_fsync"
  number_HAL_read_call7/1 -> Bus Creator4/14  "HAL_ref_IMU_temp"
  number_HAL_read_call1/1 -> Bus Creator4/2  "timestamp"
  HAL_fifo_gyro_SI_t_creator3/1(HAL_fifo_acce_SI_TempCorr) -> Bus Creator4/13  "HAL_fifo_acce_SI"
  HAL_acc_SI_creator/1(HAL_acc_SI) -> Bus Creator4/6  "HAL_acc_SI"
  HAL_fifo_gyro_SI_t_creator/1(HAL_fifo_gyro_SI_TempCorr) -> Bus Creator4/10  "HAL_fifo_gyro_SI_TempCorr"
  Demux3/3 -> HAL_acc_SI_creator/3(z)  "z"
  HAL_pressure_SI_creator/1(HAL_pressure_SI) -> Bus Creator4/18  "HAL_pressure_SI"
  Bus Creator4/1 -> HAL_acquisition_t/1  "HAL_acquisition_t"
  HAL_ultrasound_SI_creator/1(HAL_ultrasound_SI) -> Bus Creator4/19  "HAL_ultrasound_SI"

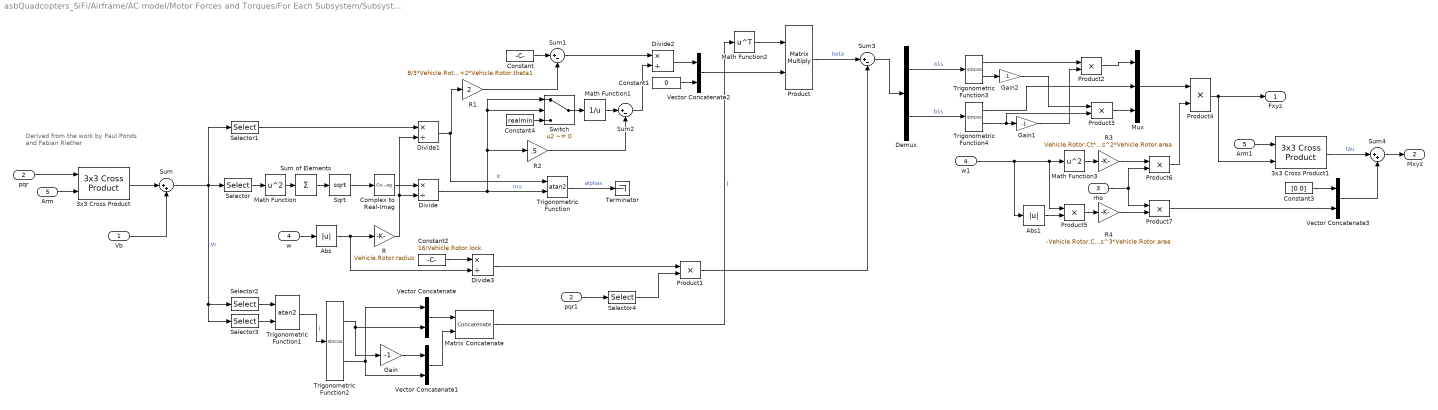
== system asbQuadcopters_SiFi/Airframe/AC model/Motor Forces and Torques/For Each Subsystem/Subsystem ==
  note: Derived from the work by Paul Ponds
      | and Fabian Riether
  Vb : Inport  PortDimensions=3
  pqr : Inport  Port=2  PortDimensions=3
  rho : Inport  Port=3  PortDimensions=1
  w : Inport  Port=4  PortDimensions=[1 1]
  Arm : Inport  Port=5  PortDimensions=[3 1]
  3x3 Cross Product : sharedutil/3x3 Cross Product  aMode=aMode
      settings: SourceProductBaseCode=AE
  3x3 Cross Product1 : sharedutil/3x3 Cross Product  aMode=aMode
      settings: SourceProductBaseCode=AE
  Abs : Abs
  Abs1 : Abs
  Arm1 : InportShadow  Port=5  PortDimensions=[3 1]
  Complex to Real-Imag : ComplexToRealImag  Output=Real
  Constant : Constant  Value=8/3*Vehicle.Rotor.theta0+2*Vehicle.Rotor.theta1
  Constant1 : Constant  Value=0
  Constant2 : Constant  Value=16/Vehicle.Rotor.lock
  Constant3 : Constant  Value=[0 0]
  Constant4 : Constant  Value=realmin
  Demux : Demux  Outputs=2
  Divide{,1..3} (4 alike) : Product  Inputs=*/
  Gain : Gain  Gain=-1
  Gain1 : Gain  Gain=-1
  Gain2 : Gain  Gain=-1
  Math Function : Math  Operator=square  SaturateOnIntegerOverflow=on
  Math Function1 : Math  Operator=reciprocal  SaturateOnIntegerOverflow=on
  Math Function2 : Math  Operator=transpose  SaturateOnIntegerOverflow=on
  Math Function3 : Math  Operator=square  SaturateOnIntegerOverflow=on
  Matrix Concatenate : Concatenate  Mode=Multidimensional array  ConcatenateDimension=2
  Mux : Mux  Inputs=3
  Product : Product  Multiplication=Matrix(*)
  Product{1..7} (7 alike) : Product
  R : Gain  Gain=Vehicle.Rotor.radius
  R1 : Gain  Gain=2
  R2 : Gain  Gain=.5
  R3 : Gain  Gain=Vehicle.Rotor.Ct*Vehicle.Rotor.radius^2*Vehicle.Rotor.area
  R4 : Gain  Gain=-Vehicle.Rotor.Cq*Vehicle.Rotor.radius^3*Vehicle.Rotor.area
  Selector : Selector  InputPortWidth=3  IndexOptions=Index vector (dialog)  Indices=[1 2]  OutputSizes=1
  Selector1 : Selector  InputPortWidth=3  IndexOptions=Index vector (dialog)  Indices=[3]  OutputSizes=1
  Selector2 : Selector  InputPortWidth=3  IndexOptions=Index vector (dialog)  Indices=[2]  OutputSizes=1
  Selector3 : Selector  InputPortWidth=3  IndexOptions=Index vector (dialog)  Indices=[1]  OutputSizes=1
  Selector4 : Selector  InputPortWidth=3  IndexOptions=Index vector (dialog)  Indices=[2 1]  OutputSizes=1
  Sqrt : Sqrt  OutputSignalType=complex  SaturateOnIntegerOverflow=on
  Sum : Sum  Inputs=|++
  Sum of Elements : Sum  Inputs=+
  Sum1 : Sum  Inputs=|+-
  Sum2 : Sum  Inputs=|+-
  Sum3 : Sum  Inputs=|+-
  Sum4 : Sum  Inputs=|++
  Switch : Switch  Criteria=u2 ~= 0
  Terminator : Terminator
  Trigonometric Function : Trigonometry  Operator=atan2
  Trigonometric Function1 : Trigonometry  Operator=atan2
  Trigonometric Function2 : Trigonometry  Operator=sincos
  Trigonometric Function3 : Trigonometry  Operator=sincos
  Trigonometric Function4 : Trigonometry  Operator=sincos
  Vector Concatenate{,1..3} (4 alike) : Concatenate
  pqr1 : InportShadow  Port=2  PortDimensions=3
  w1 : InportShadow  Port=4  PortDimensions=[1 1]
  Fxyz : Outport  PortDimensions=[3 1]
  Mxyz : Outport  Port=2  PortDimensions=[3 1]
  wires:
  Product4/1 -> Fxyz/1, 3x3 Cross Product1/2
  3x3 Cross Product/1 -> Sum/1
  Matrix Concatenate/1 -> Math Function2/1  "J"
  Divide1/1 -> Trigonometric Function/1, R1/1  "lc"
  w/1 -> Abs/1
  Product7/1 -> Vector Concatenate3/2
  Sum/1 -> Selector/1, Selector1/1, Selector2/1, Selector3/1  "Vr"
  Abs/1 -> R/1, Divide3/2
  Math Function1/1 -> Sum2/1
  R2/1 -> Sum2/2
  Selector1/1 -> Divide1/1
  Selector/1 -> Math Function/1
  R/1 -> Divide/2, Divide1/2
  Arm/1 -> 3x3 Cross Product/2
  pqr/1 -> 3x3 Cross Product/1
  Product2/1 -> Mux/1
  Trigonometric Function3/2 -> Gain2/1
  Vector Concatenate/1 -> Matrix Concatenate/1
  Gain1/1 -> Product2/2
  Vector Concatenate1/1 -> Matrix Concatenate/2
  Sum2/1 -> Divide2/2
  Trigonometric Function2/1 -> Gain/1, Vector Concatenate/2
  Sum1/1 -> Divide2/1
  Trigonometric Function3/1 -> Product2/1
  Constant1/1 -> Vector Concatenate2/2
  3x3 Cross Product1/1 -> Sum4/1  "tau"
  Math Function3/1 -> R3/1
  Demux/2 -> Trigonometric Function4/1  "b1s"
  Trigonometric Function2/2 -> Vector Concatenate/1, Vector Concatenate1/2
  pqr1/1 -> Selector4/1
  Gain/1 -> Vector Concatenate1/1
  Selector3/1 -> Trigonometric Function1/2
  Selector2/1 -> Trigonometric Function1/1
  Product3/1 -> Mux/3
  R1/1 -> Sum1/2
  Trigonometric Function1/1 -> Trigonometric Function2/1  "j"
  Constant2/1 -> Divide3/1
  Sum of Elements/1 -> Sqrt/1
  Trigonometric Function/1 -> Terminator/1  "alphas"
  Constant/1 -> Sum1/1
  Divide3/1 -> Product1/1
  Selector4/1 -> Product1/2
  Abs1/1 -> Product5/2
  Product/1 -> Sum3/1  "beta"
  Vector Concatenate2/1 -> Product/2
  Divide2/1 -> Vector Concatenate2/1
  Product6/1 -> Product4/2
  Trigonometric Function4/1 -> Mux/2
  Mux/1 -> Product4/1
  Vb/1 -> Sum/2
  Vector Concatenate3/1 -> Sum4/2
  R4/1 -> Product7/2
  Divide/1 -> Trigonometric Function/2, Switch/1, Switch/2, R2/1  "mu"
  Complex to Real-Imag/1 -> Divide/1
  Math Function2/1 -> Product/1
  Sum4/1 -> Mxyz/1
  Math Function/1 -> Sum of Elements/1
  Demux/1 -> Trigonometric Function3/1  "a1s"
  Gain2/1 -> Product3/1
  Sum3/1 -> Demux/1
  Switch/1 -> Math Function1/1
  Product5/1 -> R4/1
  Product1/1 -> Sum3/2
  Constant3/1 -> Vector Concatenate3/1
  Trigonometric Function4/2 -> Gain1/1, Product3/2
  w1/1 -> Math Function3/1, Product5/1, Abs1/1
  rho/1 -> Product7/1, Product6/2
  Constant4/1 -> Switch/3
  Arm1/1 -> 3x3 Cross Product1/1
  Sqrt/1 -> Complex to Real-Imag/1
  R3/1 -> Product6/1

== system asbQuadcopters_SiFi/FCS/State Estimator/EstimatorXYPosition/EstimatorVelocity/AccelerationHandling ==
  dxy_estimin : Inport
  sensorIMU_datin : Inport  Port=2
  orient_estimin : Inport  Port=3
  Z_estimin : Inport  Port=4
  Add : Sum  Inputs=-+
  Bus Selector1 : BusSelector  OutputSignals=ddx,ddy,ddz
  Deactivate Acceleration If OF is not used due to low altitude : simulink/Logic and Bit Operations/Compare To Constant  relop=<=  const=Estimator.pos.opticalFlowZMax  OutDataTypeStr=boolean
  Logical Operator : Logic  Operator=OR  AllPortsSameDT=off  OutDataTypeStr=boolean
  Mux6 : Mux  Inputs=3
  Product : Product  Inputs=3
  Product1 : Product  Multiplication=Matrix(*)
  Rotation Angles to Direction Cosine Matrix : sharedtransform/Rotation Angles to Direction Cosine Matrix  rotationOrder=ZYX  aMode=aMode
      settings: SourceProductBaseCode=AE
  SelectPlanarddxy : Selector  InputPortWidth=3  IndexOptions=Index vector (dialog)  Indices=[1 2]  OutputSizes=1
  Selector : Selector  InputPortWidth=2  IndexOptions=Index vector (dialog)  Indices=1  OutputSizes=1
  Selector1 : Selector  InputPortWidth=2  IndexOptions=Index vector (dialog)  Indices=2  OutputSizes=1
  do not use acc if optical flow never available (Note OF@60Hz but ZOH to 200!) : simulink/Logic and Bit Operations/Compare To Constant  relop=~=  const=0  OutDataTypeStr=boolean
  do not use acc if optical flow never available (Note OF@60Hz but ZOH to 200!)1 : simulink/Logic and Bit Operations/Compare To Constant  relop=~=  const=0  OutDataTypeStr=boolean
  gainaccinput : Gain  Gain=Estimator.pos.accelerationInputGain  OutDataTypeStr=single
  gravity : Constant  Value=[0 0 -g]
  acceleration_world : Outport  OutDataTypeStr=single
  wires:
  do not use acc if optical flow never available (Note OF@60Hz but ZOH to 200!)1/1 -> Logical Operator/2
  do not use acc if optical flow never available (Note OF@60Hz but ZOH to 200!)/1 -> Logical Operator/1
  Logical Operator/1 -> Product/1
  Selector1/1 -> do not use acc if optical flow never available (Note OF@60Hz but ZOH to 200!)1/1
  Selector/1 -> do not use acc if optical flow never available (Note OF@60Hz but ZOH to 200!)/1
  dxy_estimin/1 -> Selector1/1, Selector/1
  Product/1 -> acceleration_world/1
  Deactivate Acceleration If OF is not used due to low altitude/1 -> Product/3
  Z_estimin/1 -> Deactivate Acceleration If OF is not used due to low altitude/1
  Add/1 -> SelectPlanarddxy/1
  Product1/1 -> Add/1
  gravity/1 -> Product1/2
  gainaccinput/1 -> Product/2
  SelectPlanarddxy/1 -> gainaccinput/1
  Bus Selector1/3 -> Mux6/3  "<ddz>"
  Bus Selector1/1 -> Mux6/1  "<ddx>"
  sensorIMU_datin/1 -> Bus Selector1/1
  Mux6/1 -> Add/2
  Bus Selector1/2 -> Mux6/2  "<ddy>"
  orient_estimin/1 -> Rotation Angles to Direction Cosine Matrix/1
  Rotation Angles to Direction Cosine Matrix/1 -> Product1/1

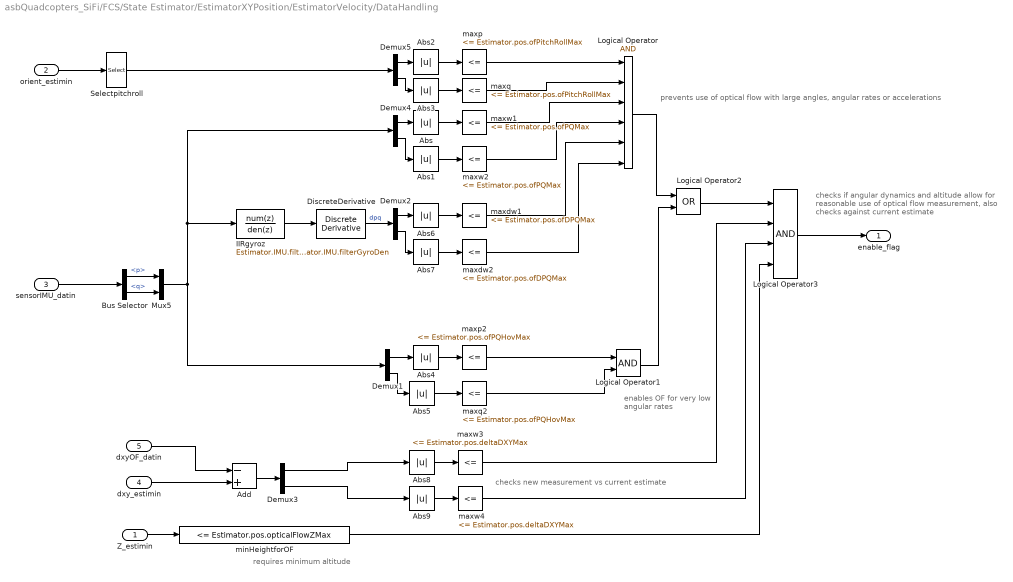
== system asbQuadcopters_SiFi/FCS/State Estimator/EstimatorXYPosition/EstimatorVelocity/DataHandling ==
  note: prevents use of optical flow with large angles, angular rates or accelerations
  note: enables OF for very
      | low angular rates
  note: checks if angular dynamics and altitude allow for
      | reasonable use of optical flow measurement,
      | also checks against current estimate
  note: checks new measurement vs current estimate
  note: requires minimum altitude
  Z_estimin : Inport
  orient_estimin : Inport  Port=2
  sensorIMU_datin : Inport  Port=3
  dxy_estimin : Inport  Port=4
  dxyOF_datin : Inport  Port=5
  Abs{,1..9} (10 alike) : Abs
  Add : Sum  Inputs=-+
  Bus Selector : BusSelector  OutputSignals=p,q
  Demux{1..5} (5 alike) : Demux  Outputs=2
  DiscreteDerivative : simulink/Discrete/Discrete Derivative  gainval=1.0  ICPrevScaledInput=0.0  InputProcessing=Inherited  OutMin=[]  OutMax=[]  OutDataType=fixdt(1, 16)  OutScaling=2^-10  DoSatur=off
  IIRgyroz : DiscreteFilter  Numerator=Estimator.IMU.filterGyroNum  Denominator=Estimator.IMU.filterGyroDen
  Logical Operator : Logic  Inputs=6  AllPortsSameDT=off  OutDataTypeStr=boolean
  Logical Operator1 : Logic  AllPortsSameDT=off  OutDataTypeStr=boolean
  Logical Operator2 : Logic  Operator=OR  AllPortsSameDT=off  OutDataTypeStr=boolean
  Logical Operator3 : Logic  Inputs=4  AllPortsSameDT=off  OutDataTypeStr=boolean
  Mux5 : Mux  Inputs=2
  Selectpitchroll : Selector  InputPortWidth=3  IndexOptions=Index vector (dialog)  Indices=[2 3]  OutputSizes=1
  maxdw1 : simulink/Logic and Bit Operations/Compare To Constant  relop=<=  const=Estimator.pos.ofDPQMax  OutDataTypeStr=boolean
  maxdw2 : simulink/Logic and Bit Operations/Compare To Constant  relop=<=  const=Estimator.pos.ofDPQMax  OutDataTypeStr=boolean
  maxp : simulink/Logic and Bit Operations/Compare To Constant  relop=<=  const=Estimator.pos.ofPitchRollMax  OutDataTypeStr=boolean
  maxp2 : simulink/Logic and Bit Operations/Compare To Constant  relop=<=  const=Estimator.pos.ofPQHovMax  OutDataTypeStr=boolean
  maxq : simulink/Logic and Bit Operations/Compare To Constant  relop=<=  const=Estimator.pos.ofPitchRollMax  OutDataTypeStr=boolean
  maxq2 : simulink/Logic and Bit Operations/Compare To Constant  relop=<=  const=Estimator.pos.ofPQHovMax  OutDataTypeStr=boolean
  maxw1 : simulink/Logic and Bit Operations/Compare To Constant  relop=<=  const=Estimator.pos.ofPQMax  OutDataTypeStr=boolean
  maxw2 : simulink/Logic and Bit Operations/Compare To Constant  relop=<=  const=Estimator.pos.ofPQMax  OutDataTypeStr=boolean
  maxw3 : simulink/Logic and Bit Operations/Compare To Constant  relop=<=  const=Estimator.pos.deltaDXYMax  OutDataTypeStr=boolean
  maxw4 : simulink/Logic and Bit Operations/Compare To Constant  relop=<=  const=Estimator.pos.deltaDXYMax  OutDataTypeStr=boolean
  minHeightforOF : simulink/Logic and Bit Operations/Compare To Constant  relop=<=  const=Estimator.pos.opticalFlowZMax  OutDataTypeStr=boolean
  enable_flag : Outport
  wires:
  minHeightforOF/1 -> Logical Operator3/4
  IIRgyroz/1 -> DiscreteDerivative/1
  Mux5/1 -> Demux1/1, IIRgyroz/1, Demux4/1
  maxw4/1 -> Logical Operator3/3
  maxw3/1 -> Logical Operator3/2
  dxyOF_datin/1 -> Add/1
  Demux3/2 -> Abs9/1
  Demux3/1 -> Abs8/1
  dxy_estimin/1 -> Add/2
  Add/1 -> Demux3/1
  Abs9/1 -> maxw4/1
  Abs8/1 -> maxw3/1
  Logical Operator2/1 -> Logical Operator3/1
  Logical Operator3/1 -> enable_flag/1
  DiscreteDerivative/1 -> Demux2/1  "dpq"
  Demux2/2 -> Abs7/1
  Demux2/1 -> Abs6/1
  Abs7/1 -> maxdw2/1
  Abs6/1 -> maxdw1/1
  Logical Operator1/1 -> Logical Operator2/2
  Demux1/2 -> Abs5/1
  Demux1/1 -> Abs4/1
  Abs5/1 -> maxq2/1
  Abs4/1 -> maxp2/1
  Abs3/1 -> maxq/1
  Abs2/1 -> maxp/1
  Demux4/2 -> Abs1/1
  Demux4/1 -> Abs/1
  Abs1/1 -> maxw2/1
  Abs/1 -> maxw1/1
  Z_estimin/1 -> minHeightforOF/1
  Logical Operator/1 -> Logical Operator2/1
  maxw1/1 -> Logical Operator/3
  Bus Selector/1 -> Mux5/1  "<p>"
  Selectpitchroll/1 -> Demux5/1
  sensorIMU_datin/1 -> Bus Selector/1
  maxq2/1 -> Logical Operator1/2
  Bus Selector/2 -> Mux5/2  "<q>"
  maxp/1 -> Logical Operator/1
  maxw2/1 -> Logical Operator/4
  orient_estimin/1 -> Selectpitchroll/1
  maxdw1/1 -> Logical Operator/5
  maxdw2/1 -> Logical Operator/6
  maxq/1 -> Logical Operator/2
  Demux5/1 -> Abs2/1
  Demux5/2 -> Abs3/1
  maxp2/1 -> Logical Operator1/1

== system asbQuadcopters_SiFi/FCS/State Estimator/EstimatorXYPosition/EstimatorXYPosition/OutlierHandling ==
  orient_estimin : Inport
  posVIS_datin : Inport  Port=2
  pos_estim : Inport  Port=3
  Abs : Abs
  Abs1 : Abs
  Add1 : Sum  Inputs=+-  AccumDataTypeStr=single
  Constant : Constant  Value=2  OutDataTypeStr=single
  Demux : Demux  Outputs=2
  Logical Operator3 : Logic  Inputs=4  AllPortsSameDT=off  OutDataTypeStr=boolean
  Math Function : Math  Operator=pow  SaturateOnIntegerOverflow=on
  SelectX : Selector  InputPortWidth=4  IndexOptions=Index vector (dialog)  Indices=[1]  OutputSizes=1
  SelectXY : Selector  InputPortWidth=4  IndexOptions=Index vector (dialog)  Indices=[1 2]  OutputSizes=1
  Selector : Selector  InputPortWidth=3  IndexOptions=Index vector (dialog)  Indices=[2 3]  OutputSizes=1
  Sqrt : Sqrt  SaturateOnIntegerOverflow=on
  Sum of Elements : Sum  Inputs=+
  checkifPosavailable : simulink/Logic and Bit Operations/Compare To Constant  relop=~=  const=-99  OutDataTypeStr=boolean
  maxp3 : simulink/Logic and Bit Operations/Compare To Constant  relop=<=  const=Estimator.pos.visOrientMax  OutDataTypeStr=boolean
  maxq3 : simulink/Logic and Bit Operations/Compare To Constant  relop=<=  const=Estimator.pos.visOrientMax  OutDataTypeStr=boolean
  planarjumpsVISPOS : simulink/Logic and Bit Operations/Compare To Constant  relop=<  const=Estimator.pos.visDeltaXYMax  OutDataTypeStr=boolean
  enable_flag : Outport
  wires:
  Abs1/1 -> maxq3/1
  Abs/1 -> maxp3/1
  Demux/2 -> Abs1/1
  Demux/1 -> Abs/1
  Selector/1 -> Demux/1
  orient_estimin/1 -> Selector/1
  planarjumpsVISPOS/1 -> Logical Operator3/4
  Sqrt/1 -> planarjumpsVISPOS/1
  pos_estim/1 -> Add1/2
  Add1/1 -> Math Function/1
  SelectXY/1 -> Add1/1
  maxq3/1 -> Logical Operator3/3
  maxp3/1 -> Logical Operator3/2
  Logical Operator3/1 -> enable_flag/1
  checkifPosavailable/1 -> Logical Operator3/1
  SelectX/1 -> checkifPosavailable/1
  posVIS_datin/1 -> SelectX/1, SelectXY/1
  Sum of Elements/1 -> Sqrt/1
  Constant/1 -> Math Function/2
  Math Function/1 -> Sum of Elements/1

== system asbQuadcopters_SiFi/Sensor/Sensor System/IMU_Pressure/HAL_acquisition_creator/HAL_acc_SI_creator ==
  x : Inport
  y : Inport  Port=2
  z : Inport  Port=3
  Bus Creator : BusCreator  Inputs=4  OutDataTypeStr=Bus: HAL_acc_SI_t
  temperature : Constant  Value=0  OutDataTypeStr=single
  HAL_acc_SI : Outport
  wires:
  temperature/1 -> Bus Creator/4  "temperature"
  Bus Creator/1 -> HAL_acc_SI/1  "HAL_acc_SI"
  x/1 -> Bus Creator/1
  y/1 -> Bus Creator/2
  z/1 -> Bus Creator/3
